simulink model "gm_wahWahEffect"  (R2022b)
settings: Solver=FixedStepDiscrete  StartTime=0.0  StopTime=simParams.stopTime  RelTol=1e-3
PostLoadFcn:
  | postLoadCallback
InitFcn:
  | initCallback
StopFcn:
  | stopCallback
undefined symbols (not defined in the file or in its folder): modelParams
libraries: dspsigops x11, dspsrcs4 x8, hdlmdlgenlib x2
(part 1 of 2)
settings Model: PacingRate=0.110000  Creator=foruf  LastModifiedBy=Sohai
settings DataIOCC: ReturnWorkspaceOutputs=off
settings OptimizationCC: BlockReduction=off  ConditionallyExecuteInputs=off  DefaultParameterBehavior=Inlined  InheritOutputTypeSmallerThanSingle=on
settings DebuggingCC: AlgebraicLoopMsg=error  InheritedTsInSrcMsg=none  SingleTaskRateTransMsg=error  ParameterPrecisionLossMsg=none
settings HardwareCC: ProdBitPerPointer=32  ProdBitPerSizeT=32  ProdBitPerPtrDiffT=32  ProdLargestAtomicFloat=None  ProdIntDivRoundTo=Undefined  ProdEndianess=Unspecified  ProdWordSize=32  ProdHWDeviceType=ASIC/FPGA->ASIC/FPGA  TargetBitPerPointer=64  TargetBitPerSizeT=64  TargetBitPerPtrDiffT=64  TargetLongLongMode=on  TargetIntDivRoundTo=Zero  TargetEndianess=LittleEndian  TargetWordSize=64  TargetHWDeviceType=Custom Processor->MATLAB Host Computer  ProdEqTarget=off
settings ModelReferenceCC: EnableRefExpFcnMdlSchedulingChecks=on

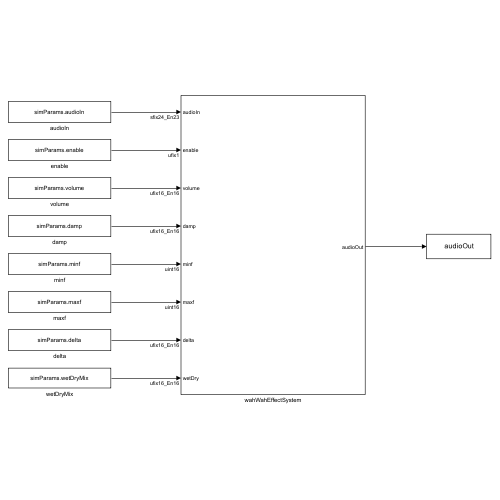
[thumbnail: Simulink's stored preview of the top-level diagram]
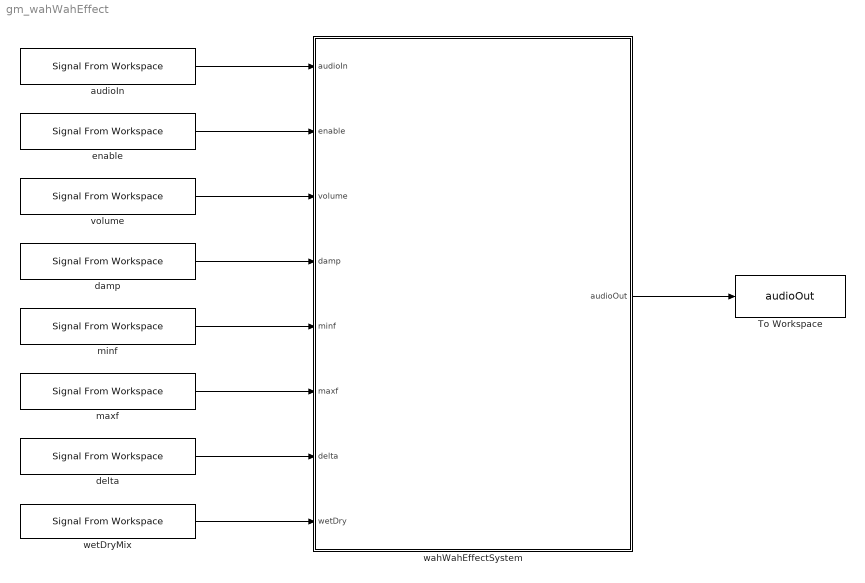
== system gm_wahWahEffect ==
  To Workspace : ToWorkspace  VariableName=audioOut  SampleTime=-1
      settings: Save2DSignal=2-D array (concatenate along first dimension)
  audioIn : dspsrcs4/Signal From Workspace  X=simParams.audioIn  Ts=modelParams.audio.samplePeriod  nsamps=1  OutputAfterFinalValue=Setting to zero  ignoreOrWarnInputAndFrameLengths=off  OutputFrames=off
  damp : dspsrcs4/Signal From Workspace  X=simParams.damp  Ts=modelParams.audio.samplePeriod  nsamps=1  OutputAfterFinalValue=Holding final value  ignoreOrWarnInputAndFrameLengths=off  OutputFrames=off
  delta : dspsrcs4/Signal From Workspace  X=simParams.delta  Ts=modelParams.audio.samplePeriod  nsamps=1  OutputAfterFinalValue=Holding final value  ignoreOrWarnInputAndFrameLengths=off  OutputFrames=off
  enable : dspsrcs4/Signal From Workspace  X=simParams.enable  Ts=modelParams.audio.samplePeriod  nsamps=1  OutputAfterFinalValue=Holding final value  ignoreOrWarnInputAndFrameLengths=off  OutputFrames=off
  maxf : dspsrcs4/Signal From Workspace  X=simParams.maxf  Ts=modelParams.audio.samplePeriod  nsamps=1  OutputAfterFinalValue=Holding final value  ignoreOrWarnInputAndFrameLengths=off  OutputFrames=off
  minf : dspsrcs4/Signal From Workspace  X=simParams.minf  Ts=modelParams.audio.samplePeriod  nsamps=1  OutputAfterFinalValue=Holding final value  ignoreOrWarnInputAndFrameLengths=off  OutputFrames=off
  volume : dspsrcs4/Signal From Workspace  X=simParams.volume  Ts=modelParams.audio.samplePeriod  nsamps=1  OutputAfterFinalValue=Holding final value  ignoreOrWarnInputAndFrameLengths=off  OutputFrames=off
  wahWahEffectSystem : Subsystem
  wetDryMix : dspsrcs4/Signal From Workspace  X=simParams.wetDryMix  Ts=modelParams.audio.samplePeriod  nsamps=1  OutputAfterFinalValue=Holding final value  ignoreOrWarnInputAndFrameLengths=off  OutputFrames=off
  wires:
  wetDryMix/1 -> wahWahEffectSystem/8(wetDry)
  delta/1 -> wahWahEffectSystem/7(delta)
  maxf/1 -> wahWahEffectSystem/6(maxf)
  minf/1 -> wahWahEffectSystem/5(minf)
  wahWahEffectSystem/1(audioOut) -> To Workspace/1
  damp/1 -> wahWahEffectSystem/4(damp)
  volume/1 -> wahWahEffectSystem/3(volume)
  enable/1 -> wahWahEffectSystem/2(enable)
  audioIn/1 -> wahWahEffectSystem/1(audioIn)

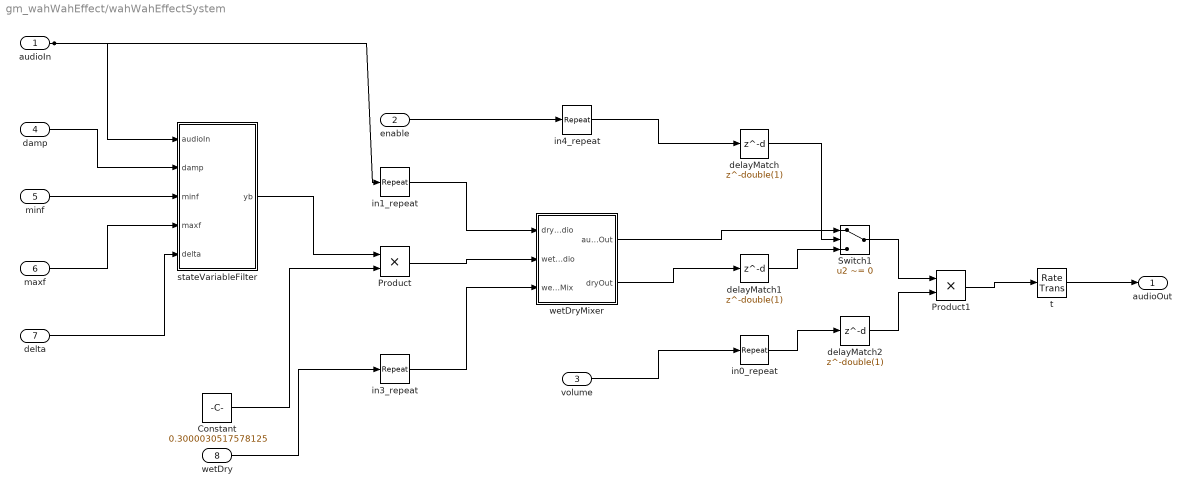
== system gm_wahWahEffect/wahWahEffectSystem ==
  audioIn : Inport  OutDataTypeStr=fixdt(1, 24, 23)  PortDimensions=1  SampleTime=2.08333333333333e-05
  enable : Inport  Port=2  OutDataTypeStr=fixdt(0, 1, 0)  PortDimensions=1  SampleTime=2.08333333333333e-05
  volume : Inport  Port=3  OutMin=[0]  OutDataTypeStr=fixdt(0, 16, 16)  PortDimensions=1  SampleTime=2.08333333333333e-05
  damp : Inport  Port=4  OutMin=[0]  OutDataTypeStr=fixdt(0, 16, 16)  PortDimensions=1  SampleTime=2.08333333333333e-05
  minf : Inport  Port=5  OutMin=[0]  OutDataTypeStr=uint16  PortDimensions=1  SampleTime=2.08333333333333e-05
  maxf : Inport  Port=6  OutMin=[0]  OutDataTypeStr=uint16  PortDimensions=1  SampleTime=2.08333333333333e-05
  delta : Inport  Port=7  OutMin=[0]  OutDataTypeStr=fixdt(0, 16, 16)  PortDimensions=1  SampleTime=2.08333333333333e-05
  wetDry : Inport  Port=8  OutDataTypeStr=fixdt(0, 16, 16)  PortDimensions=1  SampleTime=2.08333333333333e-05
  Constant : Constant  Value=0.3000030517578125  OutDataTypeStr=fixdt(0, 16, 16)  SampleTime=1.01725260416667e-08
  Product : Product  Inputs=**  OutDataTypeStr=fixdt(1, 24, 23)  SampleTime=1.01725260416667e-08
  Product1 : Product  Inputs=**  OutDataTypeStr=fixdt(1, 24, 23)  SampleTime=1.01725260416667e-08
  Switch1 : Switch  Criteria=u2 ~= 0  Threshold=double(0)  OutDataTypeStr=fixdt(1, 43, 39)  SampleTime=1.01725260416667e-08  SaturateOnIntegerOverflow=off  InputSameDT=off
  delayMatch : Delay  DelayLength=double(1)  InitialCondition=0  SampleTime=1.01725260416667e-08
  delayMatch1 : Delay  DelayLength=double(1)  InitialCondition=0  SampleTime=1.01725260416667e-08
  delayMatch2 : Delay  DelayLength=double(1)  InitialCondition=0  SampleTime=1.01725260416667e-08
  in0_repeat : dspsigops/Repeat  N=double(2048)  RateOptions=Allow multirate processing  ic=0  mode=Unused parameter value
  in1_repeat : dspsigops/Repeat  N=double(2048)  RateOptions=Allow multirate processing  ic=0  mode=Unused parameter value
  in3_repeat : dspsigops/Repeat  N=double(2048)  RateOptions=Allow multirate processing  ic=0  mode=Unused parameter value
  in4_repeat : dspsigops/Repeat  N=double(2048)  RateOptions=Allow multirate processing  ic=0  mode=Unused parameter value
  stateVariableFilter : Subsystem
  t : RateTransition  OutPortSampleTimeOpt=Multiple of input port sample time  OutPortSampleTimeMultiple=2048
  wetDryMixer : Subsystem
  audioOut : Outport  SampleTime=2.08333333333333e-05
  wires:
  audioIn/1 -> stateVariableFilter/1(audioIn), in1_repeat/1
  enable/1 -> in4_repeat/1
  volume/1 -> in0_repeat/1
  damp/1 -> stateVariableFilter/2(damp)
  minf/1 -> stateVariableFilter/3(minf)
  maxf/1 -> stateVariableFilter/4(maxf)
  delta/1 -> stateVariableFilter/5(delta)
  wetDry/1 -> in3_repeat/1
  stateVariableFilter/1(yb) -> Product/1
  t/1 -> audioOut/1
  in0_repeat/1 -> delayMatch2/1
  in1_repeat/1 -> wetDryMixer/1(dryAudio)
  in3_repeat/1 -> wetDryMixer/3(wetDryMix)
  in4_repeat/1 -> delayMatch/1
  Product1/1 -> t/1
  Constant/1 -> Product/2
  Product/1 -> wetDryMixer/2(wetAudio)
  wetDryMixer/1(audioOut) -> Switch1/1
  delayMatch1/1 -> Switch1/3
  Switch1/1 -> Product1/1
  delayMatch2/1 -> Product1/2
  delayMatch/1 -> Switch1/2
  wetDryMixer/2(dryOut) -> delayMatch1/1

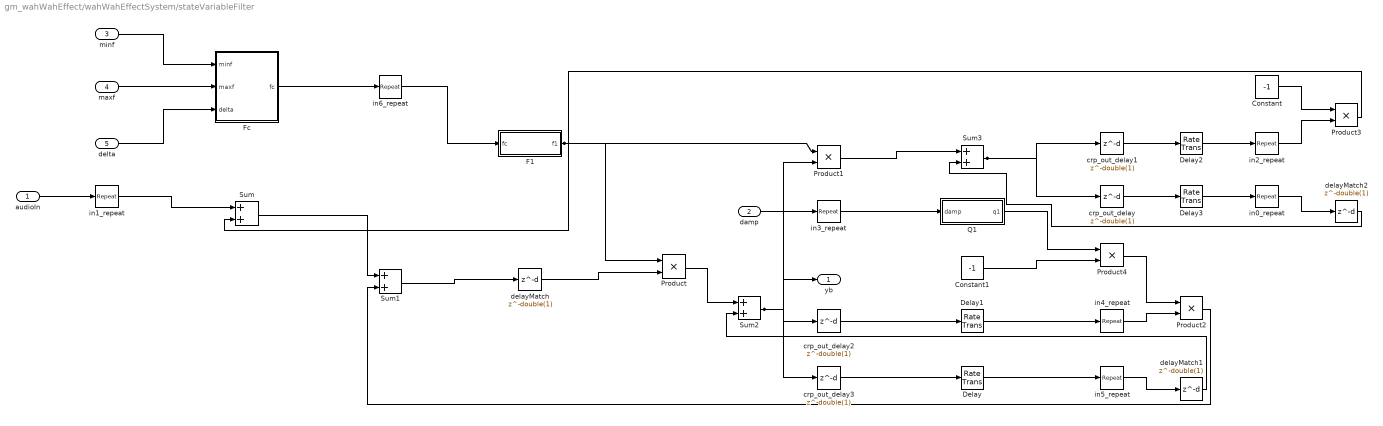
== system gm_wahWahEffect/wahWahEffectSystem/stateVariableFilter ==
  audioIn : Inport  OutDataTypeStr=fixdt(1, 24, 23)  PortDimensions=1  SampleTime=2.08333333333333e-05
  damp : Inport  Port=2  OutDataTypeStr=fixdt(0, 16, 16)  PortDimensions=1  SampleTime=2.08333333333333e-05
  minf : Inport  Port=3  OutDataTypeStr=uint16  PortDimensions=1  SampleTime=2.08333333333333e-05
  maxf : Inport  Port=4  OutDataTypeStr=uint16  PortDimensions=1  SampleTime=2.08333333333333e-05
  delta : Inport  Port=5  OutDataTypeStr=fixdt(0, 16, 16)  PortDimensions=1  SampleTime=2.08333333333333e-05
  Constant : Constant  Value=-1  OutDataTypeStr=fixdt(1, 2, 0)  SampleTime=1.01725260416667e-08
  Constant1 : Constant  Value=-1  OutDataTypeStr=fixdt(1, 2, 0)  SampleTime=1.01725260416667e-08
  Delay{,1..3} (4 alike) : RateTransition  OutPortSampleTimeOpt=Multiple of input port sample time  OutPortSampleTimeMultiple=2048
  F1 : Subsystem
  Fc : Subsystem
  Product{,1..4} (5 alike) : Product  Inputs=**  OutDataTypeStr=fixdt(1, 69, 48)  SampleTime=1.01725260416667e-08
  Q1 : Subsystem
  Sum : Sum  AccumDataTypeStr=fixdt(1, 70, 48)  OutDataTypeStr=fixdt(1, 70, 48)  SaturateOnIntegerOverflow=on  SampleTime=1.01725260416667e-08
  Sum1 : Sum  AccumDataTypeStr=fixdt(1, 71, 48)  OutDataTypeStr=fixdt(1, 71, 48)  SaturateOnIntegerOverflow=on  SampleTime=1.01725260416667e-08
  Sum2 : Sum  AccumDataTypeStr=fixdt(1, 71, 48)  OutDataTypeStr=fixdt(1, 70, 48)  SaturateOnIntegerOverflow=on  SampleTime=1.01725260416667e-08
  Sum3 : Sum  AccumDataTypeStr=fixdt(1, 70, 48)  OutDataTypeStr=fixdt(1, 69, 48)  SaturateOnIntegerOverflow=on  SampleTime=1.01725260416667e-08
  crp_out_delay{,1..3} (4 alike) : Delay  DelayLength=double(1)  InitialCondition=0  SampleTime=1.01725260416667e-08
  delayMatch : Delay  DelayLength=double(1)  InitialCondition=0  SampleTime=1.01725260416667e-08
  delayMatch1 : Delay  DelayLength=double(1)  InitialCondition=0  SampleTime=1.01725260416667e-08
  delayMatch2 : Delay  DelayLength=double(1)  InitialCondition=0  SampleTime=1.01725260416667e-08
  in0_repeat : dspsigops/Repeat  N=double(2048)  RateOptions=Allow multirate processing  ic=0  mode=Unused parameter value
  in1_repeat : dspsigops/Repeat  N=double(2048)  RateOptions=Allow multirate processing  ic=0  mode=Unused parameter value
  in2_repeat : dspsigops/Repeat  N=double(2048)  RateOptions=Allow multirate processing  ic=0  mode=Unused parameter value
  in3_repeat : dspsigops/Repeat  N=double(2048)  RateOptions=Allow multirate processing  ic=0  mode=Unused parameter value
  in4_repeat : dspsigops/Repeat  N=double(2048)  RateOptions=Allow multirate processing  ic=0  mode=Unused parameter value
  in5_repeat : dspsigops/Repeat  N=double(2048)  RateOptions=Allow multirate processing  ic=0  mode=Unused parameter value
  in6_repeat : dspsigops/Repeat  N=double(2048)  RateOptions=Allow multirate processing  ic=0  mode=Unused parameter value
  yb : Outport  SampleTime=1.01725260416667e-08
  wires:
  Fc/1(fc) -> in6_repeat/1
  Sum2/1 -> yb/1, Product1/2, crp_out_delay2/1, crp_out_delay3/1
  audioIn/1 -> in1_repeat/1
  damp/1 -> in3_repeat/1
  minf/1 -> Fc/1(minf)
  maxf/1 -> Fc/2(maxf)
  delta/1 -> Fc/3(delta)
  Delay3/1 -> in0_repeat/1
  Delay2/1 -> in2_repeat/1
  Delay1/1 -> in4_repeat/1
  Delay/1 -> in5_repeat/1
  in0_repeat/1 -> delayMatch2/1
  in1_repeat/1 -> Sum/1
  in2_repeat/1 -> Product3/2
  in3_repeat/1 -> Q1/1(damp)
  in4_repeat/1 -> Product2/2
  in5_repeat/1 -> delayMatch1/1
  in6_repeat/1 -> F1/1(fc)
  crp_out_delay/1 -> Delay3/1
  crp_out_delay1/1 -> Delay2/1
  crp_out_delay2/1 -> Delay1/1
  crp_out_delay3/1 -> Delay/1
  Sum3/1 -> crp_out_delay/1, crp_out_delay1/1
  Constant/1 -> Product3/1
  Product3/1 -> Sum/2
  Sum/1 -> Sum1/1
  Q1/1(q1) -> Product4/1
  Constant1/1 -> Product4/2
  Product4/1 -> Product2/1
  Product2/1 -> Sum1/2
  delayMatch/1 -> Product/2
  Product/1 -> Sum2/1
  Product1/1 -> Sum3/1
  F1/1(f1) -> Product1/1, Product/1
  delayMatch2/1 -> Sum3/2
  delayMatch1/1 -> Sum2/2
  Sum1/1 -> delayMatch/1

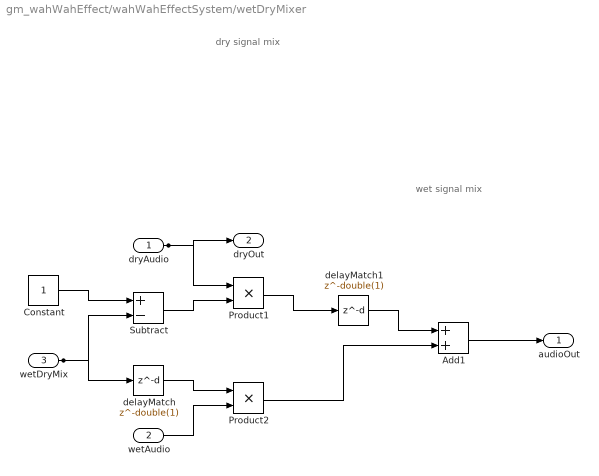
== system gm_wahWahEffect/wahWahEffectSystem/wetDryMixer ==
  note: dry signal mix
  note: wet signal mix
  dryAudio : Inport  OutDataTypeStr=fixdt(1, 24, 23)  PortDimensions=1  SampleTime=1.01725260416667e-08
  wetAudio : Inport  Port=2  OutDataTypeStr=fixdt(1, 24, 23)  PortDimensions=1  SampleTime=1.01725260416667e-08
  wetDryMix : Inport  Port=3  OutDataTypeStr=fixdt(0, 16, 16)  PortDimensions=1  SampleTime=1.01725260416667e-08
  Add1 : Sum  AccumDataTypeStr=fixdt(1, 43, 39)  OutDataTypeStr=fixdt(1, 43, 39)  SaturateOnIntegerOverflow=on  SampleTime=1.01725260416667e-08
  Constant : Constant  OutDataTypeStr=fixdt(0, 1, 0)  SampleTime=1.01725260416667e-08
  Product1 : Product  Inputs=**  OutDataTypeStr=fixdt(1, 42, 39)  SampleTime=1.01725260416667e-08
  Product2 : Product  Inputs=**  OutDataTypeStr=fixdt(1, 40, 39)  SampleTime=1.01725260416667e-08
  Subtract : Sum  Inputs=+-  AccumDataTypeStr=fixdt(1, 18, 16)  OutDataTypeStr=fixdt(1, 18, 16)  SaturateOnIntegerOverflow=on  SampleTime=1.01725260416667e-08
  delayMatch : Delay  DelayLength=double(1)  InitialCondition=0  SampleTime=1.01725260416667e-08
  delayMatch1 : Delay  DelayLength=double(1)  InitialCondition=0  SampleTime=1.01725260416667e-08
  audioOut : Outport  SampleTime=1.01725260416667e-08
  dryOut : Outport  Port=2  SampleTime=1.01725260416667e-08
  wires:
  delayMatch/1 -> Product2/1
  Add1/1 -> audioOut/1
  Constant/1 -> Subtract/1
  delayMatch1/1 -> Add1/1
  Product2/1 -> Add1/2
  Subtract/1 -> Product1/2
  Product1/1 -> delayMatch1/1
  dryAudio/1 -> Product1/1, dryOut/1
  wetAudio/1 -> Product2/2
  wetDryMix/1 -> delayMatch/1, Subtract/2

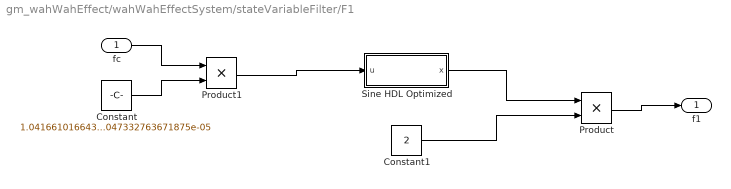
== system gm_wahWahEffect/wahWahEffectSystem/stateVariableFilter/F1 ==
  fc : Inport  OutDataTypeStr=fixdt(1, 34, 16)  PortDimensions=1  SampleTime=1.01725260416667e-08
  Constant : Constant  Value=1.041661016643047332763671875e-05  OutDataTypeStr=fixdt(0, 32, 32)  SampleTime=1.01725260416667e-08
  Constant1 : Constant  Value=2  OutDataTypeStr=fixdt(0, 2, 0)  SampleTime=1.01725260416667e-08
  Product : Product  Inputs=**  OutDataTypeStr=fixdt(1, 69, 48)  SampleTime=1.01725260416667e-08
  Product1 : Product  Inputs=**  OutDataTypeStr=fixdt(1, 66, 48)  SampleTime=1.01725260416667e-08
  Sine HDL Optimized : Subsystem  mask(Sine and Cosine HDL optimized block){OutputFormula=sin(2*pi*u), NumDataPoints=double(1024), TableDataTypeStr=fixdt(1,66,48), SimulateLUTROMDelay=off}
      mask prompts: OutputFormula "Simulink:masks:OutputFormula_MP"; NumDataPoints "HDLShared:hdlshared:CosineHDL_Npts"; TableDataTypeStr "Simulink:blkprm_prompts:TABLE_UNIFIEDDATATYPE"; SimulateLUTROMDelay "HDLShared:hdlshared:CosineHDL_SimulateLUTDelay"
      mask help: Sine and Cosine HDL optimized block using quarter wave symmetry, and HDL friendly settings.
      mask Help: helpview([docroot '/hdlcoder/helptargets.map'],'SineAndCosineHDL_Optimized');
      mask TypeOptions OutputFormula: sin(2*pi*u) | cos(2*pi*u) | exp(j*2*pi*u) | sin(2*pi*u) and cos(2*pi*u)
      mask Display:
      | port_label('input',1,'u')
      | port_label('output',1,'sin(2*pi*u)')
      | xpos = 0.35;
      | yoffset = 0.5;
      | if ( SimulateLUTROMDelay )
      |   text(xpos,yoffset,'HDL (Z^{-1})','texmode','on')
      | else
      |    text(xpos,yoffset,'HDL')
      | end
  f1 : Outport  SampleTime=1.01725260416667e-08
  wires:
  Constant/1 -> Product1/2
  Constant1/1 -> Product/2
  Product/1 -> f1/1
  Product1/1 -> Sine HDL Optimized/1(u)
  Sine HDL Optimized/1(x) -> Product/1
  fc/1 -> Product1/1

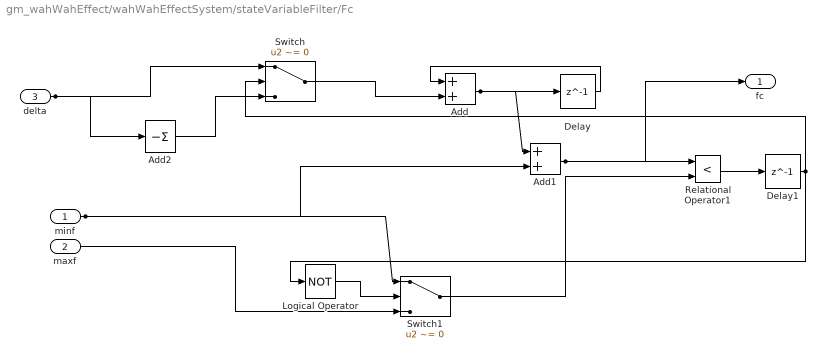
== system gm_wahWahEffect/wahWahEffectSystem/stateVariableFilter/Fc ==
  minf : Inport  OutDataTypeStr=uint16  PortDimensions=1  SampleTime=2.08333333333333e-05
  maxf : Inport  Port=2  OutDataTypeStr=uint16  PortDimensions=1  SampleTime=2.08333333333333e-05
  delta : Inport  Port=3  OutDataTypeStr=fixdt(0, 16, 16)  PortDimensions=1  SampleTime=2.08333333333333e-05
  Add : Sum  OutDataTypeStr=fixdt(1,34,16)  SaturateOnIntegerOverflow=on
  Add1 : Sum  OutDataTypeStr=fixdt(1,34,16)  SaturateOnIntegerOverflow=on
  Add2 : Sum  Inputs=-
  Delay : Delay  DelayLength=1  InitialCondition=0
  Delay1 : Delay  DelayLength=1  InitialCondition=0
  Logical Operator : Logic  Operator=NOT  AllPortsSameDT=off  OutDataTypeStr=boolean
  Relational Operator1 : RelationalOperator  Operator=<  OutDataTypeStr=boolean  InputSameDT=off
  Switch : Switch  Criteria=u2 ~= 0  SaturateOnIntegerOverflow=off  InputSameDT=off
  Switch1 : Switch  Criteria=u2 ~= 0  SaturateOnIntegerOverflow=off  InputSameDT=off
  fc : Outport  SampleTime=2.08333333333333e-05
  wires:
  Add1/1 -> fc/1, Relational Operator1/1
  Add2/1 -> Switch/3
  minf/1 -> Switch1/1, Add1/2
  maxf/1 -> Switch1/3
  delta/1 -> Switch/1, Add2/1
  Switch/1 -> Add/2
  Relational Operator1/1 -> Delay1/1
  Switch1/1 -> Relational Operator1/2
  Logical Operator/1 -> Switch1/2
  Delay1/1 -> Switch/2, Logical Operator/1
  Add/1 -> Add1/1, Delay/1
  Delay/1 -> Add/1

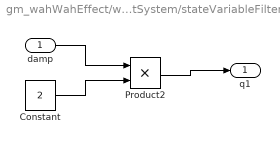
== system gm_wahWahEffect/wahWahEffectSystem/stateVariableFilter/Q1 ==
  damp : Inport  OutDataTypeStr=fixdt(0, 16, 16)  PortDimensions=1  SampleTime=1.01725260416667e-08
  Constant : Constant  Value=2  OutDataTypeStr=fixdt(0, 2, 0)  SampleTime=1.01725260416667e-08
  Product2 : Product  Inputs=**  OutDataTypeStr=fixdt(0, 18, 16)  SampleTime=1.01725260416667e-08
  q1 : Outport  SampleTime=1.01725260416667e-08
  wires:
  Constant/1 -> Product2/2
  Product2/1 -> q1/1
  damp/1 -> Product2/1
